simulink model "W06_city_highway_cs"  (R2019a)
settings: Solver=ode5  StartTime=0.0  StopTime=inf  FixedStep=1/60  RelTol=1e-3
PreLoadFcn:
  | mbxruntime.callbacks.PreLoadFcn(bdroot);
PostLoadFcn:
  | mbxruntime.callbacks.PostLoadFcn(bdroot);
InitFcn:
  | mbxruntime.callbacks.InitFcn(bdroot);
StartFcn:
  | mbxruntime.callbacks.StartFcn(bdroot);
StopFcn:
  | mbxruntime.callbacks.StopFcn(bdroot);
model workspace: external: MAT-File .\W06_city_highway_cs_hws.mat (data not in the file)
undefined symbols (not defined in the file or in its folder): DiscIntNeverNeededParam, FovAzimuth, FovAzimuthDefined, FovElevation, FovElevationDefined, Header, InitImageOutputDir, LocationX, LocationXDefined, LocationY, LocationYDefined, LocationZ, LocationZDefined, Orientation, OrientationPitch, OrientationPitchDefined, OrientationRoll, OrientationRollDefined, OrientationYaw, OrientationYawDefined, Poses, Poses_SL_Info, Position, W06_city_highway_cs_0270c22595f3b0e3, W06_city_highway_cs_086892688dd32ddc, W06_city_highway_cs_328c49ac39fca66b, W06_city_highway_cs_35ce05381b8ebe8c, W06_city_highway_cs_47b384f162638175, W06_city_highway_cs_766f76ce4de94dd5, W06_city_highway_cs_8c547f67cb81ffba, W06_city_highway_cs_aed52f2a7724a4f9, W06_city_highway_cs_Audi_A8_Sedan_1_Path_pathUniqueID, W06_city_highway_cs_b74cbb1f9f7331b5, W06_city_highway_cs_Citroen_C3_Hatchback_1_Path_pathUniqueID, W06_city_highway_cs_d395f8835e0c28b3, W06_city_highway_cs_e5f9d1759e19e2b4, W06_city_highway_cs_Toyota_Previa_MPV_1_Path_pathUniqueID
libraries: adeye_lib x26, simulink_extras x24, robotlib x7, sharedtransform x4, PreScanSimulinkLibrary x2, PreScanUsefulBlocks x1
(part 2 of 8)

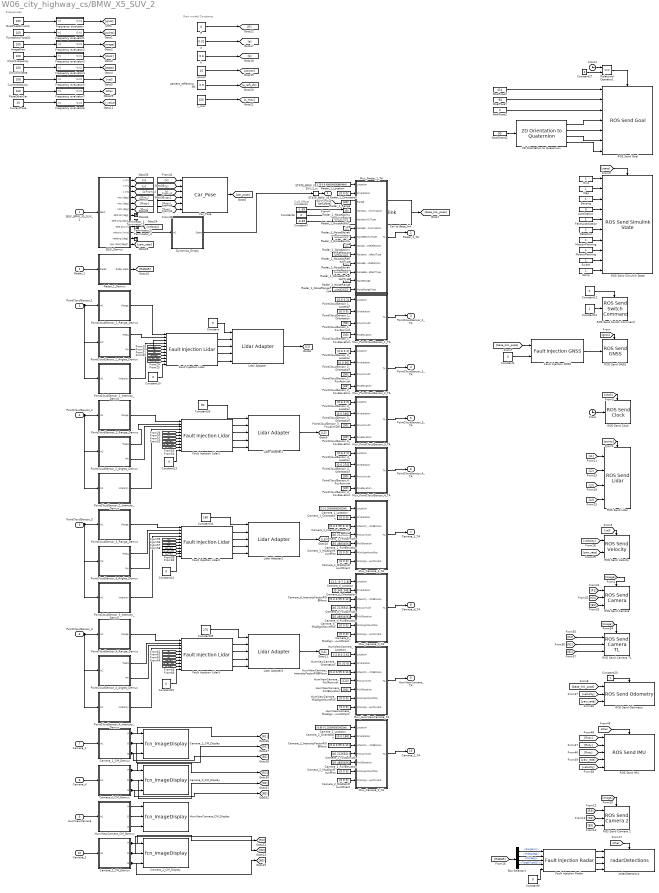
== system W06_city_highway_cs/BMW_X5_SUV_2 ==
  note: Frequencies
  note: CoG Offset
  note: Rain model Constants
  SELF_BMW_X5_SUV_2 : Inport  Tag=inport/SelfPort  OutDataTypeStr=Bus: PRESCAN_SELFSENSORDATA  PortDimensions=1  SampleTime=1/60  BusOutputAsStruct=on
  Radar_1 : Inport  Tag=inport/Radar  Port=2  OutDataTypeStr=Bus: PRESCAN_SCANNERSENSOR_MESSAGE  PortDimensions=7  SampleTime=1/20  BusOutputAsStruct=on
  PointCloudSensor_1 : Inport  Tag=inport/PointCloudInport  Port=3  OutDataTypeStr=single  SampleTime=1/20  BusOutputAsStruct=on
  PointCloudSensor_2 : Inport  Tag=inport/PointCloudInport  Port=4  OutDataTypeStr=single  SampleTime=1/20  BusOutputAsStruct=on
  PointCloudSensor_3 : Inport  Tag=inport/PointCloudInport  Port=5  OutDataTypeStr=single  SampleTime=1/20  BusOutputAsStruct=on
  PointCloudSensor_4 : Inport  Tag=inport/PointCloudInport  Port=6  OutDataTypeStr=single  SampleTime=1/20  BusOutputAsStruct=on
  Camera_1 : Inport  Tag=inport/Camera/CameraSensor  Port=7  OutDataTypeStr=uint8  SampleTime=1/20  BusOutputAsStruct=on
  Camera_tl : Inport  Tag=inport/Camera/CameraSensor  Port=8  OutDataTypeStr=uint8  SampleTime=1/20  BusOutputAsStruct=on
  HumViewCamera : Inport  Tag=inport/Camera/CameraSensor  Port=9  OutDataTypeStr=uint8  SampleTime=1/60  BusOutputAsStruct=on
  Camera_2 : Inport  Tag=inport/Camera/CameraSensor  Port=10  OutDataTypeStr=uint8  SampleTime=1/20  BusOutputAsStruct=on
  2D Orientation to Quaternion : adeye_lib/2D Orientation to Quaternion  SystemSampleTime=-1
  Bus Selector1 : BusSelector  OutputSignals=Range[m],Theta[deg],Phi[deg],TargetTypeID[-]
  Camera_1_CM_Demux : Subsystem  Tag=demux/Camera/Color  mask{SensorName=Camera_1, hres=960, vres=720}
      mask prompts: SensorName "Sensor Name"; hres "Horizontal Resolution"; vres "Vertical Resolution"
      mask Help: eval('openHelp(457)')
      mask Display:
      | fprintf('MONO CAMERA:\n Color\n %s \n %d x %d px',SensorName,hres,vres)
      | port_label('output',1,'R')
      | port_label('output',2,'G')
      | port_label('output',3,'B')
  Camera_1_CM_Display : M-S-Function  Tag=CameraSensor_Color_Display  InitFcn=InitImageOutputDir(gcb);  FunctionName=fcn_ImageDisplay  Parameters=SensorName EnableDisplay EnablePosition DisplayPosition FigureHandle SaveResults BitmapFormat TempOutputDir CameraType DataType  mask(PreScan Color Display Block){SensorName=Camera_1, EnableDisplay=on, EnablePosition=off, DisplayPosition=[10 10 960 720], FigureHandle=640605, SaveResults=off, Format=PNG, TempOutputDir=0, CameraType=Mono, DataType=uint8}
      mask prompts: SensorName "User Specified: Title of Display"; EnableDisplay "Active"; EnablePosition "Set Display window position"; DisplayPosition "Display window position [xpos ypos width height]"; FigureHandle "Unique Handle"; SaveResults "Save results"; TempOutputDir "OutputDir"; CameraType "Camera Type"; DataType "Image Data Type"
      mask help: This block displays the RGB output of a PreScan camera sensor.
      mask init:
      | if EnableDisplay
      |     EnableString='';
      |     EnableColor='gray';
      | else
      |     EnableString='INACTIVE';
      |     EnableColor='red';
      | end
      | switch Format
      |     case 1
      |         BitmapFormat = 'png';
      |     case 2
      |         BitmapFormat = 'bmp';
      |     case 3
      |         BitmapFormat = 'jpg';
      | end 
      | if CameraType==1
      |     CameraTypeName='MONO';
      |     PortNumber=0;
      | else
      |     CameraTypeName='STEREO';
      |     PortNumber=3;
      | end
      settings: CopyFcn=CopyFcnDisplay  DeleteFcn=PreScanBlockDeleteFcn;  ModelCloseFcn=fcn_ImageDisplay_ModelCloseFcn
      mask Help: eval('openHelp(457)')
      mask Callback EnablePosition:
      | MV=get_param(gcb,'MaskVisibilities');
      | if strcmp(get_param(gcb,'EnablePosition'),'on')
      |     MV{4}='on';
      | else
      |     MV{4}='off';
      | end
      | set_param(gcb,'MaskVisibilities',MV);
      | clear MV;
      mask TypeOptions Format: PNG | BMP | JPG
      mask TypeOptions CameraType: Mono | Stereo
      mask TypeOptions DataType: uint8 | single
      mask Display:
      | color(EnableColor);
      | fprintf('%s\n DISPLAY:\n Color \n %s',EnableString,SensorName)
      | port_label('input',1,'R')
      | port_label('input',2,'G')
      | port_label('input',3,'B')
      | port_label('input',PortNumber+1,'R')
      | port_label('input',PortNumber+2,'G')
      | port_label('input',PortNumber+3,'B')
  Camera_1_FoVAzimuth : Constant  Tag=Camera_1_FoVAzimuth  Value=[46.2126541]
  Camera_1_FoVElevation : Constant  Tag=Camera_1_FoVElevation  Value=[35.4893456]
  Camera_1_IntensityFactorRGBMono : Constant  Tag=Camera_1_IntensityFactorRGBMono  Value=[0.3 0.59 0.11]
  Camera_1_Location : Constant  Tag=Camera_1_Location  Value=[2 0 1.32000005245209]
  Camera_1_MisAlignMountOrient : Constant  Tag=Camera_1_MisAlignMountOrient  Value=[0 0 0]
  Camera_1_MisAlignMountPos : Constant  Tag=Camera_1_MisAlignMountPos  Value=[0 0 0]
  Camera_1_Orientation : Constant  Tag=Camera_1_Orientation  Value=[0 0 0]
  Camera_2_CM_Demux : Subsystem  Tag=demux/Camera/Color  mask{SensorName=Camera_2, hres=960, vres=720}
      mask prompts: SensorName "Sensor Name"; hres "Horizontal Resolution"; vres "Vertical Resolution"
      mask Help: eval('openHelp(457)')
      mask Display:
      | fprintf('MONO CAMERA:\n Color\n %s \n %d x %d px',SensorName,hres,vres)
      | port_label('output',1,'R')
      | port_label('output',2,'G')
      | port_label('output',3,'B')
  Camera_2_CM_Display : M-S-Function  Tag=CameraSensor_Color_Display  InitFcn=InitImageOutputDir(gcb);  FunctionName=fcn_ImageDisplay  Parameters=SensorName EnableDisplay EnablePosition DisplayPosition FigureHandle SaveResults BitmapFormat TempOutputDir CameraType DataType  mask(PreScan Color Display Block){SensorName=Camera_2, EnableDisplay=on, EnablePosition=off, DisplayPosition=[10 10 960 720], FigureHandle=640608, SaveResults=off, Format=PNG, TempOutputDir=0, CameraType=Mono, DataType=uint8}
      mask prompts: SensorName "User Specified: Title of Display"; EnableDisplay "Active"; EnablePosition "Set Display window position"; DisplayPosition "Display window position [xpos ypos width height]"; FigureHandle "Unique Handle"; SaveResults "Save results"; TempOutputDir "OutputDir"; CameraType "Camera Type"; DataType "Image Data Type"
      mask help: This block displays the RGB output of a PreScan camera sensor.
      mask init: same as W06_city_highway_cs/BMW_X5_SUV_2/Camera_1_CM_Display
      settings: CopyFcn=CopyFcnDisplay  DeleteFcn=PreScanBlockDeleteFcn;  ModelCloseFcn=fcn_ImageDisplay_ModelCloseFcn
      mask Help: eval('openHelp(457)')
      mask Callback EnablePosition:
      | MV=get_param(gcb,'MaskVisibilities');
      | if strcmp(get_param(gcb,'EnablePosition'),'on')
      |     MV{4}='on';
      | else
      |     MV{4}='off';
      | end
      | set_param(gcb,'MaskVisibilities',MV);
      | clear MV;
      mask TypeOptions Format: PNG | BMP | JPG
      mask TypeOptions CameraType: Mono | Stereo
      mask TypeOptions DataType: uint8 | single
      mask Display:
      | color(EnableColor);
      | fprintf('%s\n DISPLAY:\n Color \n %s',EnableString,SensorName)
      | port_label('input',1,'R')
      | port_label('input',2,'G')
      | port_label('input',3,'B')
      | port_label('input',PortNumber+1,'R')
      | port_label('input',PortNumber+2,'G')
      | port_label('input',PortNumber+3,'B')
  Camera_2_FoVAzimuth : Constant  Tag=Camera_2_FoVAzimuth  Value=[46.2126541]
  Camera_2_FoVElevation : Constant  Tag=Camera_2_FoVElevation  Value=[35.4893456]
  Camera_2_IntensityFactorRGBMono : Constant  Tag=Camera_2_IntensityFactorRGBMono  Value=[0.3 0.59 0.11]
  Camera_2_Location : Constant  Tag=Camera_2_Location  Value=[-0.95 0 1.32000005245209]
  Camera_2_MisAlignMountOrient : Constant  Tag=Camera_2_MisAlignMountOrient  Value=[0 0 0]
  Camera_2_MisAlignMountPos : Constant  Tag=Camera_2_MisAlignMountPos  Value=[0 0 0]
  Camera_2_Orientation : Constant  Tag=Camera_2_Orientation  Value=[0 0 180]
  Camera_tl_CM_Demux : Subsystem  Tag=demux/Camera/Color  mask{SensorName=Camera_tl, hres=960, vres=720}
      mask prompts: SensorName "Sensor Name"; hres "Horizontal Resolution"; vres "Vertical Resolution"
      mask Help: eval('openHelp(457)')
      mask Display:
      | fprintf('MONO CAMERA:\n Color\n %s \n %d x %d px',SensorName,hres,vres)
      | port_label('output',1,'R')
      | port_label('output',2,'G')
      | port_label('output',3,'B')
  Camera_tl_CM_Display : M-S-Function  Tag=CameraSensor_Color_Display  InitFcn=InitImageOutputDir(gcb);  FunctionName=fcn_ImageDisplay  Parameters=SensorName EnableDisplay EnablePosition DisplayPosition FigureHandle SaveResults BitmapFormat TempOutputDir CameraType DataType  mask(PreScan Color Display Block){SensorName=Camera_tl, EnableDisplay=on, EnablePosition=off, DisplayPosition=[10 10 960 720], FigureHandle=640606, SaveResults=off, Format=PNG, TempOutputDir=0, CameraType=Mono, DataType=uint8}
      mask prompts: SensorName "User Specified: Title of Display"; EnableDisplay "Active"; EnablePosition "Set Display window position"; DisplayPosition "Display window position [xpos ypos width height]"; FigureHandle "Unique Handle"; SaveResults "Save results"; TempOutputDir "OutputDir"; CameraType "Camera Type"; DataType "Image Data Type"
      mask help: This block displays the RGB output of a PreScan camera sensor.
      mask init: same as W06_city_highway_cs/BMW_X5_SUV_2/Camera_1_CM_Display
      settings: CopyFcn=CopyFcnDisplay  DeleteFcn=PreScanBlockDeleteFcn;  ModelCloseFcn=fcn_ImageDisplay_ModelCloseFcn
      mask Help: eval('openHelp(457)')
      mask Callback EnablePosition:
      | MV=get_param(gcb,'MaskVisibilities');
      | if strcmp(get_param(gcb,'EnablePosition'),'on')
      |     MV{4}='on';
      | else
      |     MV{4}='off';
      | end
      | set_param(gcb,'MaskVisibilities',MV);
      | clear MV;
      mask TypeOptions Format: PNG | BMP | JPG
      mask TypeOptions CameraType: Mono | Stereo
      mask TypeOptions DataType: uint8 | single
      mask Display:
      | color(EnableColor);
      | fprintf('%s\n DISPLAY:\n Color \n %s',EnableString,SensorName)
      | port_label('input',1,'R')
      | port_label('input',2,'G')
      | port_label('input',3,'B')
      | port_label('input',PortNumber+1,'R')
      | port_label('input',PortNumber+2,'G')
      | port_label('input',PortNumber+3,'B')
  Camera_tl_FoVAzimuth : Constant  Tag=Camera_tl_FoVAzimuth  Value=[46.2126541]
  Camera_tl_FoVElevation : Constant  Tag=Camera_tl_FoVElevation  Value=[35.4893456]
  Camera_tl_IntensityFactorRGBMono : Constant  Tag=Camera_tl_IntensityFactorRGBMono  Value=[0.3 0.59 0.11]
  Camera_tl_Location : Constant  Tag=Camera_tl_Location  Value=[1.1 -0.7 1.8]
  Camera_tl_MisAlignMountOrient : Constant  Tag=Camera_tl_MisAlignMountOrient  Value=[0 0 0]
  Camera_tl_MisAlignMountPos : Constant  Tag=Camera_tl_MisAlignMountPos  Value=[0 0 0]
  Camera_tl_Orientation : Constant  Tag=Camera_tl_Orientation  Value=[0 345 345]
  Car to Base_link : adeye_lib/Car to Base_link  SystemSampleTime=-1
  Car_Pose : adeye_lib/Car_Pose  SystemSampleTime=-1
  Clock : Clock
  Clock2 : Clock
  ClockFrequency : Constant  Value=100
  Constant{,10,13..15} (5 alike) : Constant  Value=0  OutDataTypeStr=Inherit: Inherit via back propagation
  Constant1 : Constant  Value=0  OutDataTypeStr=Inherit: Inherit via back propagation  SampleTime=0.05
  Constant11 : Constant  OutDataTypeStr=Inherit: Inherit via back propagation  SampleTime=0.05
  Constant12 : Constant  Value=0  OutDataTypeStr=Inherit: Inherit via back propagation  SampleTime=0.05
  Constant2 : Constant  Value=-1.69
  Constant20 : Constant
  Constant27 : Constant  Value=0
  Constant33 : Constant  Value=90  OutDataTypeStr=Inherit: Inherit via back propagation
  Constant34 : Constant  Value=180  OutDataTypeStr=Inherit: Inherit via back propagation
  Constant35 : Constant  Value=270  OutDataTypeStr=Inherit: Inherit via back propagation
  Constant6 : Constant  Value=0
  Constant7 : Constant  Value=-0.69
  Constant9 : Constant  Value=0
  CurrentPose : Constant  Value=10
  CurrentVelocity : Constant  Value=100
  Detection : Constant
  Dynamics_Empty : Subsystem  Tag=Dynamics_Empty
      mask Help: eval('openHelp(202)')
      mask Display: port_label('output', 1, 'State');text(0,0,' Empty\n')
  FakeLocalization : Constant
  Fault Injection GNSS : adeye_lib/Fault Injection GNSS  v=0.0001  f=20
  Fault Injection Lidar{,1..3} (4 alike) : adeye_lib/Fault Injection Lidar  vr=0.0001  vi=0.0001  f=20  p=225*16
  Fault Injection Radar : adeye_lib/Fault Injection Radar  n=7  vr=1  vt=1  vp=1
  Frequency evaluator : Subsystem
  Frequency evaluator1 : Subsystem
  Frequency evaluator2 : Subsystem
  Frequency evaluator3 : Subsystem
  Frequency evaluator4 : Subsystem
  Frequency evaluator5 : Subsystem
  Frequency evaluator6 : Subsystem
  Frequency evaluator7 : Subsystem
  GnssPoseSimulink : Constant  Value=100
  GoalOrientZ : Constant  Value=90
  GoalPoseX : Constant  Value=414
  GoalPoseY : Constant  Value=-83
  GoalPoseZ : Constant  Value=0
  HumViewCamera_CM_Demux : Subsystem  Tag=demux/Camera/Color  mask{SensorName=HumViewCamera, hres=1871, vres=1080}
      mask prompts: SensorName "Sensor Name"; hres "Horizontal Resolution"; vres "Vertical Resolution"
      mask Help: eval('openHelp(457)')
      mask Display:
      | fprintf('MONO CAMERA:\n Color\n %s \n %d x %d px',SensorName,hres,vres)
      | port_label('output',1,'R')
      | port_label('output',2,'G')
      | port_label('output',3,'B')
  HumViewCamera_CM_Display : M-S-Function  Tag=CameraSensor_Color_Display  InitFcn=InitImageOutputDir(gcb);  FunctionName=fcn_ImageDisplay  Parameters=SensorName EnableDisplay EnablePosition DisplayPosition FigureHandle SaveResults BitmapFormat TempOutputDir CameraType DataType  mask(PreScan Color Display Block){SensorName=HumViewCamera, EnableDisplay=on, EnablePosition=off, DisplayPosition=[10 10 1871 1080], FigureHandle=640607, SaveResults=off, Format=PNG, TempOutputDir=0, CameraType=Mono, DataType=uint8}
      mask prompts: SensorName "User Specified: Title of Display"; EnableDisplay "Active"; EnablePosition "Set Display window position"; DisplayPosition "Display window position [xpos ypos width height]"; FigureHandle "Unique Handle"; SaveResults "Save results"; TempOutputDir "OutputDir"; CameraType "Camera Type"; DataType "Image Data Type"
      mask help: This block displays the RGB output of a PreScan camera sensor.
      mask init: same as W06_city_highway_cs/BMW_X5_SUV_2/Camera_1_CM_Display
      settings: CopyFcn=CopyFcnDisplay  DeleteFcn=PreScanBlockDeleteFcn;  ModelCloseFcn=fcn_ImageDisplay_ModelCloseFcn
      mask Help: eval('openHelp(457)')
      mask Callback EnablePosition:
      | MV=get_param(gcb,'MaskVisibilities');
      | if strcmp(get_param(gcb,'EnablePosition'),'on')
      |     MV{4}='on';
      | else
      |     MV{4}='off';
      | end
      | set_param(gcb,'MaskVisibilities',MV);
      | clear MV;
      mask TypeOptions Format: PNG | BMP | JPG
      mask TypeOptions CameraType: Mono | Stereo
      mask TypeOptions DataType: uint8 | single
      mask Display:
      | color(EnableColor);
      | fprintf('%s\n DISPLAY:\n Color \n %s',EnableString,SensorName)
      | port_label('input',1,'R')
      | port_label('input',2,'G')
      | port_label('input',3,'B')
      | port_label('input',PortNumber+1,'R')
      | port_label('input',PortNumber+2,'G')
      | port_label('input',PortNumber+3,'B')
  HumViewCamera_FoVAzimuth : Constant  Tag=HumViewCamera_FoVAzimuth  Value=[120]
  HumViewCamera_FoVElevation : Constant  Tag=HumViewCamera_FoVElevation  Value=[90]
  HumViewCamera_IntensityFactorRGBMono : Constant  Tag=HumViewCamera_IntensityFactorRGBMono  Value=[0.3 0.59 0.11]
  HumViewCamera_Location : Constant  Tag=HumViewCamera_Location  Value=[-2.8 0 2.6]
  HumViewCamera_MisAlignMountOrient : Constant  Tag=HumViewCamera_MisAlignMountOrient  Value=[0 0 0]
  HumViewCamera_MisAlignMountPos : Constant  Tag=HumViewCamera_MisAlignMountPos  Value=[0 0 0]
  HumViewCamera_Orientation : Constant  Tag=HumViewCamera_Orientation  Value=[0 31 0]
  ImageRaw : Constant  Value=100
  Lidar Adapter{,1..3} (4 alike) : adeye_lib/Lidar Adapter  SystemSampleTime=-1
  Localization : Constant  Value=0
  Map : Constant
  MissionPlanning : Constant
  MotionPlanning : Constant
  Mux_Camera_1_TA : Subsystem  Tag=mux/Camera_TA/CameraSensor
  Mux_Camera_2_TA : Subsystem  Tag=mux/Camera_TA/CameraSensor
  Mux_Camera_tl_TA : Subsystem  Tag=mux/Camera_TA/CameraSensor
  Mux_HumViewCamera_TA : Subsystem  Tag=mux/Camera_TA/CameraSensor
  Mux_PointCloudSensor_1_TA : Subsystem  Tag=mux/SensorTA
  Mux_PointCloudSensor_2_TA : Subsystem  Tag=mux/SensorTA
  Mux_PointCloudSensor_3_TA : Subsystem  Tag=mux/SensorTA
  Mux_PointCloudSensor_4_TA : Subsystem  Tag=mux/SensorTA
  Mux_Radar_1_TA : Subsystem  Tag=mux/Radar_TA
  PointCloudSensor_1_Angles_Demux : Subsystem  Tag=demux/PCS/Angles  mask{SensorName=PointCloudSensor_1, offset=225, hres=225, vres=16}
      mask prompts: SensorName "Sensor Name"; offset "Data Start"; hres "Horizontal Resolution"; vres "Vertical Resolution"
      mask Help: eval('openHelp(6400)')
      mask Display:
      | fprintf('Point Cloud:\n Data\n %s \n %d x %d px',SensorName,hres,vres)
      | port_label('output',1,'Theta')
      | port_label('output',2,'Phi')
  PointCloudSensor_1_FovAzimuth : Constant  Tag=PointCloudSensor_1_FovAzimuth  Value=[90]
  PointCloudSensor_1_FovElevation : Constant  Tag=PointCloudSensor_1_FovElevation  Value=[30]
  PointCloudSensor_1_Intensity_Demux : Subsystem  Tag=demux/PCS/Intensity  mask{SensorName=PointCloudSensor_1, offset=675, hres=225, vres=16}
      mask prompts: SensorName "Sensor Name"; offset "Data Start"; hres "Horizontal Resolution"; vres "Vertical Resolution"
      mask Help: eval('openHelp(6400)')
      mask Display:
      | fprintf('Point Cloud:\n Data\n %s \n %d x %d px',SensorName,hres,vres)
      | port_label('output',1,'Intensity')
  PointCloudSensor_1_Location : Constant  Tag=PointCloudSensor_1_Location  Value=[0.6 0 2]
  PointCloudSensor_1_Orientation : Constant  Tag=PointCloudSensor_1_Orientation  Value=[0 0 0]
  PointCloudSensor_1_Range_Demux : Subsystem  Tag=demux/PCS/Range  mask{SensorName=PointCloudSensor_1, offset=0, hres=225, vres=16}
      mask prompts: SensorName "Sensor Name"; offset "Data Start"; hres "Horizontal Resolution"; vres "Vertical Resolution"
      mask Help: eval('openHelp(6400)')
      mask Display:
      | fprintf('Point Cloud:\n Data\n %s \n %d x %d px',SensorName,hres,vres)
      | port_label('output',1,'Range')
  PointCloudSensor_2_Angles_Demux : Subsystem  Tag=demux/PCS/Angles  mask{SensorName=PointCloudSensor_2, offset=225, hres=225, vres=16}
      mask prompts: SensorName "Sensor Name"; offset "Data Start"; hres "Horizontal Resolution"; vres "Vertical Resolution"
      mask Help: eval('openHelp(6400)')
      mask Display:
      | fprintf('Point Cloud:\n Data\n %s \n %d x %d px',SensorName,hres,vres)
      | port_label('output',1,'Theta')
      | port_label('output',2,'Phi')
  PointCloudSensor_2_FovAzimuth : Constant  Tag=PointCloudSensor_2_FovAzimuth  Value=[90]
  PointCloudSensor_2_FovElevation : Constant  Tag=PointCloudSensor_2_FovElevation  Value=[30]
  PointCloudSensor_2_Intensity_Demux : Subsystem  Tag=demux/PCS/Intensity  mask{SensorName=PointCloudSensor_2, offset=675, hres=225, vres=16}
      mask prompts: SensorName "Sensor Name"; offset "Data Start"; hres "Horizontal Resolution"; vres "Vertical Resolution"
      mask Help: eval('openHelp(6400)')
      mask Display:
      | fprintf('Point Cloud:\n Data\n %s \n %d x %d px',SensorName,hres,vres)
      | port_label('output',1,'Intensity')
  PointCloudSensor_2_Location : Constant  Tag=PointCloudSensor_2_Location  Value=[0.6 0 2]
  PointCloudSensor_2_Orientation : Constant  Tag=PointCloudSensor_2_Orientation  Value=[0 0 90]
  PointCloudSensor_2_Range_Demux : Subsystem  Tag=demux/PCS/Range  mask{SensorName=PointCloudSensor_2, offset=0, hres=225, vres=16}
      mask prompts: SensorName "Sensor Name"; offset "Data Start"; hres "Horizontal Resolution"; vres "Vertical Resolution"
      mask Help: eval('openHelp(6400)')
      mask Display:
      | fprintf('Point Cloud:\n Data\n %s \n %d x %d px',SensorName,hres,vres)
      | port_label('output',1,'Range')
  PointCloudSensor_3_Angles_Demux : Subsystem  Tag=demux/PCS/Angles  mask{SensorName=PointCloudSensor_3, offset=225, hres=225, vres=16}
      mask prompts: SensorName "Sensor Name"; offset "Data Start"; hres "Horizontal Resolution"; vres "Vertical Resolution"
      mask Help: eval('openHelp(6400)')
      mask Display:
      | fprintf('Point Cloud:\n Data\n %s \n %d x %d px',SensorName,hres,vres)
      | port_label('output',1,'Theta')
      | port_label('output',2,'Phi')
  PointCloudSensor_3_FovAzimuth : Constant  Tag=PointCloudSensor_3_FovAzimuth  Value=[90]
  PointCloudSensor_3_FovElevation : Constant  Tag=PointCloudSensor_3_FovElevation  Value=[30]
  PointCloudSensor_3_Intensity_Demux : Subsystem  Tag=demux/PCS/Intensity  mask{SensorName=PointCloudSensor_3, offset=675, hres=225, vres=16}
      mask prompts: SensorName "Sensor Name"; offset "Data Start"; hres "Horizontal Resolution"; vres "Vertical Resolution"
      mask Help: eval('openHelp(6400)')
      mask Display:
      | fprintf('Point Cloud:\n Data\n %s \n %d x %d px',SensorName,hres,vres)
      | port_label('output',1,'Intensity')
  PointCloudSensor_3_Location : Constant  Tag=PointCloudSensor_3_Location  Value=[0.6 0 2]
  PointCloudSensor_3_Orientation : Constant  Tag=PointCloudSensor_3_Orientation  Value=[0 0 180]
  PointCloudSensor_3_Range_Demux : Subsystem  Tag=demux/PCS/Range  mask{SensorName=PointCloudSensor_3, offset=0, hres=225, vres=16}
      mask prompts: SensorName "Sensor Name"; offset "Data Start"; hres "Horizontal Resolution"; vres "Vertical Resolution"
      mask Help: eval('openHelp(6400)')
      mask Display:
      | fprintf('Point Cloud:\n Data\n %s \n %d x %d px',SensorName,hres,vres)
      | port_label('output',1,'Range')
  PointCloudSensor_4_Angles_Demux : Subsystem  Tag=demux/PCS/Angles  mask{SensorName=PointCloudSensor_4, offset=225, hres=225, vres=16}
      mask prompts: SensorName "Sensor Name"; offset "Data Start"; hres "Horizontal Resolution"; vres "Vertical Resolution"
      mask Help: eval('openHelp(6400)')
      mask Display:
      | fprintf('Point Cloud:\n Data\n %s \n %d x %d px',SensorName,hres,vres)
      | port_label('output',1,'Theta')
      | port_label('output',2,'Phi')
  PointCloudSensor_4_FovAzimuth : Constant  Tag=PointCloudSensor_4_FovAzimuth  Value=[90]
  PointCloudSensor_4_FovElevation : Constant  Tag=PointCloudSensor_4_FovElevation  Value=[30]
  PointCloudSensor_4_Intensity_Demux : Subsystem  Tag=demux/PCS/Intensity  mask{SensorName=PointCloudSensor_4, offset=675, hres=225, vres=16}
      mask prompts: SensorName "Sensor Name"; offset "Data Start"; hres "Horizontal Resolution"; vres "Vertical Resolution"
      mask Help: eval('openHelp(6400)')
      mask Display:
      | fprintf('Point Cloud:\n Data\n %s \n %d x %d px',SensorName,hres,vres)
      | port_label('output',1,'Intensity')
  PointCloudSensor_4_Location : Constant  Tag=PointCloudSensor_4_Location  Value=[0.6 0 2]
  PointCloudSensor_4_Orientation : Constant  Tag=PointCloudSensor_4_Orientation  Value=[0 0 270]
  PointCloudSensor_4_Range_Demux : Subsystem  Tag=demux/PCS/Range  mask{SensorName=PointCloudSensor_4, offset=0, hres=225, vres=16}
      mask prompts: SensorName "Sensor Name"; offset "Data Start"; hres "Horizontal Resolution"; vres "Vertical Resolution"
      mask Help: eval('openHelp(6400)')
      mask Display:
      | fprintf('Point Cloud:\n Data\n %s \n %d x %d px',SensorName,hres,vres)
      | port_label('output',1,'Range')
  PointsRawFloat32 : Constant  Value=100
  PoseOtherCar : Constant  Value=100
  R : Constant  Value=0
  ROS Send Camera : adeye_lib/ROS Send Camera  SystemSampleTime=-1
  ROS Send Camera 2 : adeye_lib/ROS Send Camera 2  SystemSampleTime=-1
  ROS Send Camera TL : adeye_lib/ROS Send Camera TL  SystemSampleTime=-1
  ROS Send Clock : adeye_lib/ROS Send Clock  SystemSampleTime=-1
  ROS Send GNSS : adeye_lib/ROS Send GNSS  SystemSampleTime=-1
  ROS Send Goal : adeye_lib/ROS Send Goal  SystemSampleTime=-1
  ROS Send IMU : adeye_lib/ROS Send IMU  SystemSampleTime=-1
  ROS Send Lidar : adeye_lib/ROS Send Lidar  SystemSampleTime=-1
  ROS Send Odometry : adeye_lib/ROS Send Odometry  SystemSampleTime=-1
  ROS Send Simulink State : adeye_lib/ROS Send Simulink State  SystemSampleTime=-1
  ROS Send Switch Command : adeye_lib/ROS Send Switch Command  SystemSampleTime=-1
  ROS Send Velocity : adeye_lib/ROS Send Velocity  SystemSampleTime=-1
  Radar_1_Demux : Subsystem  Tag=demux/Radar  TreatAsAtomicUnit=on  mask(PreScan Demux Block: Radar){MAXMESSAGES=7}
      mask prompts: MAXMESSAGES "Number of Objects"
      mask help:
      | The Radar Sensor is a detailed sensor based on a physical radar
      | model that includes Antenna GAIN Maps (AGM) and atmospheric
      | attenuation.
      |
      | For more information, please click Help.
      mask Help: eval('openHelp(1464)')
      mask Display:
      | port_label('input',1,'Radar')
      | port_label('output',1,'Radar Data')
  Radar_1_Location : Constant  Tag=Radar_1_Location  Value=[3.75 0 0.400000005960464]
  Radar_1_NoiseAziIlluType : Constant  Tag=Radar_1_NoiseAziIlluType  Value=uint32([0])
  Radar_1_NoiseAziReflectType : Constant  Tag=Radar_1_NoiseAziReflectType  Value=uint32([0])
  Radar_1_NoiseAzimuthIllumination : Constant  Tag=Radar_1_NoiseAzimuthIllumination  Value=[0]
  Radar_1_NoiseAzimuthReflection : Constant  Tag=Radar_1_NoiseAzimuthReflection  Value=[0]
  Radar_1_NoiseElevIlluType : Constant  Tag=Radar_1_NoiseElevIlluType  Value=uint32([0])
  Radar_1_NoiseElevReflectType : Constant  Tag=Radar_1_NoiseElevReflectType  Value=uint32([0])
  Radar_1_NoiseElevationIllumination : Constant  Tag=Radar_1_NoiseElevationIllumination  Value=[0]
  Radar_1_NoiseElevationReflection : Constant  Tag=Radar_1_NoiseElevationReflection  Value=[0]
  Radar_1_NoiseRange : Constant  Tag=Radar_1_NoiseRange  Value=[0]
  Radar_1_NoiseRangeType : Constant  Tag=Radar_1_NoiseRangeType  Value=uint32([1])
  Radar_1_Orientation : Constant  Tag=Radar_1_Orientation  Value=[0 0 0]
  Radar_1_Range : Constant  Tag=Radar_1_Range  Value=[30]
  Relational Operator1 : RelationalOperator  Operator===  OutDataTypeStr=boolean  RndMeth=Simplest
  Rviz : Constant
  SELF_Demux : Subsystem  Tag=demux/SelfPort  mask(PreScan Demux Block:){}
      mask help:
      | The SELF port shows (state) information of the actor itself. The outputs are position in the experiment's axis system and the GPS coordinates, and the object's absolute velocity and compass heading.
      |
      | For more information, please click Help.
      settings: DeleteFcn=PreScanBlockDeleteFcn;
      mask Help: eval('openHelp(462)')
      mask Display:
      | port_label('output',1,'x [m]')
      | port_label('output',2,'y [m]')
      | port_label('output',3,'z [m]','texmode','on')
      | port_label('output',4,'Rotx [deg]','texmode','on')
      | port_label('output',5,'Roty [deg]','texmode','on')
      | port_label('output',6,'Rotz [deg]','texmode','on')
      | port_label('output',7,'GPS lat [deg]','texmode','on')
      | port_label('output',8,'GPS long [deg]','texmode','on')
      | port_label('output',9,'GPS alt [m]','texmode','on')
      | port_label('output',10,'Velocity [m/s]')
      | port_label('output',11,'Heading [deg]')
      | port_label('output',12,'Yaw rate [deg/s]')
  STATE_BMW_X5_SUV_2_rc : RateTransition  Tag=mux_rc/StatePort  OutPortSampleTimeOpt=Inherit
  Sensing : Constant
  SimulinkState : Constant  Value=100
  Ssmp : Constant
  Switch : Constant
  Terminator_{1..4} (4 alike) : Terminator
  a : Constant  Value=0.01
  b : Constant  Value=0.6
  percent_reflecting_sfc : Constant  Value=0.9
  power : Constant  Value=15
  radarDetections : adeye_lib/radarDetections  SystemSampleTime=-1
  z_max : Constant  Value=150
  STATE_BMW_X5_SUV_2_bus : Outport  Tag=outport/StatePort  OutDataTypeStr=Bus: PRESCAN_STATEACTUATORDATA  PortDimensions=1  SampleTime=1/60
  Radar_1_TA : Outport  Tag=outport/Radar_TA  Port=2  OutDataTypeStr=Bus: PRESCAN_SCANNERSENSOR_TA  PortDimensions=1  SampleTime=1/60
  PointCloudSensor_1_TA : Outport  Tag=outport/SensorTA  Port=3  OutDataTypeStr=Bus: PRESCAN_PCS_TA_DATA  PortDimensions=1  SampleTime=1/60
  PointCloudSensor_2_TA : Outport  Tag=outport/SensorTA  Port=4  OutDataTypeStr=Bus: PRESCAN_PCS_TA_DATA  PortDimensions=1  SampleTime=1/60
  PointCloudSensor_3_TA : Outport  Tag=outport/SensorTA  Port=5  OutDataTypeStr=Bus: PRESCAN_PCS_TA_DATA  PortDimensions=1  SampleTime=1/60
  PointCloudSensor_4_TA : Outport  Tag=outport/SensorTA  Port=6  OutDataTypeStr=Bus: PRESCAN_PCS_TA_DATA  PortDimensions=1  SampleTime=1/60
  Camera_1_TA : Outport  Tag=outport/Camera_TA/CameraSensor  Port=7  OutDataTypeStr=Bus: PRESCAN_CAMERASENSOR_TA  PortDimensions=1  SampleTime=1/60
  Camera_tl_TA : Outport  Tag=outport/Camera_TA/CameraSensor  Port=8  OutDataTypeStr=Bus: PRESCAN_CAMERASENSOR_TA  PortDimensions=1  SampleTime=1/60
  HumViewCamera_TA : Outport  Tag=outport/Camera_TA/CameraSensor  Port=9  OutDataTypeStr=Bus: PRESCAN_CAMERASENSOR_TA  PortDimensions=1  SampleTime=1/60
  Camera_2_TA : Outport  Tag=outport/Camera_TA/CameraSensor  Port=10  OutDataTypeStr=Bus: PRESCAN_CAMERASENSOR_TA  PortDimensions=1  SampleTime=1/60
  tag scope: other=global, x_value=global
  wires:
  Camera_1_CM_Demux/1(R) -> [R1], Camera_1_CM_Display/1
  Camera_1_CM_Demux/2(G) -> [G1], Camera_1_CM_Display/2
  Camera_1_CM_Demux/3(B) -> [B1], Camera_1_CM_Display/3
  Camera_tl_CM_Demux/1(R) -> [R2], Camera_tl_CM_Display/1
  Camera_tl_CM_Demux/2(G) -> [G2], Camera_tl_CM_Display/2
  Camera_tl_CM_Demux/3(B) -> [B2], Camera_tl_CM_Display/3
  Camera_2_CM_Demux/1(R) -> [R3], Camera_2_CM_Display/1
  Camera_2_CM_Demux/2(G) -> [G3], Camera_2_CM_Display/2
  Camera_2_CM_Demux/3(B) -> [B3], Camera_2_CM_Display/3
  Radar_1_Demux/1(Radar Data) -> [RADAR]
  SELF_Demux/1(x [m]) -> [x]
  SELF_Demux/2(y [m]) -> [y]
  SELF_Demux/3(z [m]) -> [z]
  SELF_Demux/4(rotx [deg]) -> [Rotx]
  SELF_Demux/5(roty [deg]) -> [Roty]
  SELF_Demux/6(rotz [deg]) -> [Rotz]
  SELF_Demux/12(yaw rate [deg/s]) -> [yaw_rate]
  ClockFrequency/1 -> Frequency evaluator3/1(In1)
  Frequency evaluator5/1(Out1) -> [vel]
  CurrentPose/1 -> Frequency evaluator6/1(In1)
  PoseOtherCar/1 -> Frequency evaluator7/1(In1)
  PointsRawFloat32/1 -> Frequency evaluator1/1(In1)
  Frequency evaluator3/1(Out1) -> [clock]
  Frequency evaluator6/1(Out1) -> [x_value]
  SimulinkState/1 -> Frequency evaluator4/1(In1)
  Frequency evaluator1/1(Out1) -> [points]
  ImageRaw/1 -> Frequency evaluator2/1(In1)
  GnssPoseSimulink/1 -> Frequency evaluator/1(In1)
  Frequency evaluator2/1(Out1) -> [image]
  Frequency evaluator4/1(Out1) -> [state]
  CurrentVelocity/1 -> Frequency evaluator5/1(In1)
  Frequency evaluator7/1(Out1) -> [other]
  Frequency evaluator/1(Out1) -> [gnss]
  [z] -> Car_Pose/3
  [Roty] -> Car_Pose/5
  [Rotx] -> Car_Pose/4
  [y] -> Car_Pose/2
  [Rotz] -> Car_Pose/6
  [x] -> Car_Pose/1
  Car_Pose/1 -> [car_pose]
  SELF_Demux/10(velocity [m/s]) -> [velocity], Dynamics_Empty/1(In1)
  PointCloudSensor_1_Range_Demux/1(Range) -> Fault Injection Lidar/1
  PointCloudSensor_1_Angles_Demux/1(Theta) -> Fault Injection Lidar/2
  PointCloudSensor_1_Angles_Demux/2(Phi) -> Fault Injection Lidar/3
  PointCloudSensor_1_Intensity_Demux/1(Intensity) -> Fault Injection Lidar/4
  [b] -> Fault Injection Lidar/7
  [p_refl_sfc] -> Fault Injection Lidar/9
  [power] -> Fault Injection Lidar/8
  [a] -> Fault Injection Lidar/6
  Constant10/1 -> Fault Injection Lidar/11
  [z_max] -> Fault Injection Lidar/10
  [R] -> Fault Injection Lidar/5
  Fault Injection Lidar/2 -> Lidar Adapter/3
  Fault Injection Lidar/3 -> Lidar Adapter/4
  Fault Injection Lidar/1 -> Lidar Adapter/2
  Lidar Adapter/1 -> [L1]
  Fault Injection Lidar/4 -> Lidar Adapter/5
  Constant/1 -> Lidar Adapter/1
  Fault Injection Lidar1/3 -> Lidar Adapter1/4
  [z_max] -> Fault Injection Lidar1/10
  [power] -> Fault Injection Lidar1/8
  Constant33/1 -> Lidar Adapter1/1
  Fault Injection Lidar1/1 -> Lidar Adapter1/2
  [R] -> Fault Injection Lidar1/5
  [a] -> Fault Injection Lidar1/6
  Constant13/1 -> Fault Injection Lidar1/11
  [p_refl_sfc] -> Fault Injection Lidar1/9
  [b] -> Fault Injection Lidar1/7
  PointCloudSensor_2_Angles_Demux/1(Theta) -> Fault Injection Lidar1/2
  PointCloudSensor_2_Angles_Demux/2(Phi) -> Fault Injection Lidar1/3
  Fault Injection Lidar1/4 -> Lidar Adapter1/5
  Lidar Adapter1/1 -> [L2]
  PointCloudSensor_2_Intensity_Demux/1(Intensity) -> Fault Injection Lidar1/4
  PointCloudSensor_2_Range_Demux/1(Range) -> Fault Injection Lidar1/1
  Fault Injection Lidar1/2 -> Lidar Adapter1/3
  Fault Injection Lidar2/3 -> Lidar Adapter2/4
  Fault Injection Lidar2/1 -> Lidar Adapter2/2
  [b] -> Fault Injection Lidar2/7
  Constant14/1 -> Fault Injection Lidar2/11
  [z_max] -> Fault Injection Lidar2/10
  [R] -> Fault Injection Lidar2/5
  PointCloudSensor_3_Angles_Demux/1(Theta) -> Fault Injection Lidar2/2
  [p_refl_sfc] -> Fault Injection Lidar2/9
  PointCloudSensor_3_Intensity_Demux/1(Intensity) -> Fault Injection Lidar2/4
  Constant34/1 -> Lidar Adapter2/1
  [a] -> Fault Injection Lidar2/6
  [power] -> Fault Injection Lidar2/8
  PointCloudSensor_3_Range_Demux/1(Range) -> Fault Injection Lidar2/1
  Lidar Adapter2/1 -> [L3]
  Fault Injection Lidar2/4 -> Lidar Adapter2/5
  Fault Injection Lidar2/2 -> Lidar Adapter2/3
  PointCloudSensor_3_Angles_Demux/2(Phi) -> Fault Injection Lidar2/3
  Lidar Adapter3/1 -> [L4]
  Fault Injection Lidar3/1 -> Lidar Adapter3/2
  [z_max] -> Fault Injection Lidar3/10
  [power] -> Fault Injection Lidar3/8
  [b] -> Fault Injection Lidar3/7
  Fault Injection Lidar3/2 -> Lidar Adapter3/3
  Fault Injection Lidar3/3 -> Lidar Adapter3/4
  Fault Injection Lidar3/4 -> Lidar Adapter3/5
  Constant15/1 -> Fault Injection Lidar3/11
  PointCloudSensor_4_Angles_Demux/1(Theta) -> Fault Injection Lidar3/2
  Constant35/1 -> Lidar Adapter3/1
  [R] -> Fault Injection Lidar3/5
  PointCloudSensor_4_Angles_Demux/2(Phi) -> Fault Injection Lidar3/3
  [p_refl_sfc] -> Fault Injection Lidar3/9
  PointCloudSensor_4_Intensity_Demux/1(Intensity) -> Fault Injection Lidar3/4
  [a] -> Fault Injection Lidar3/6
  PointCloudSensor_4_Range_Demux/1(Range) -> Fault Injection Lidar3/1
  Constant6/1 -> Car to Base_link/3
  [car_pose] -> Car to Base_link/1
  Constant7/1 -> Car to Base_link/4
  Car to Base_link/1 -> [base_link_pose]
  Constant2/1 -> Car to Base_link/2
  z_max/1 -> [z_max]
  power/1 -> [power]
  percent_reflecting_sfc/1 -> [p_refl_sfc]
  a/1 -> [a]
  b/1 -> [b]
  R/1 -> [R]
  [state] -> ROS Send Simulink State/Enable
  GoalPoseY/1 -> ROS Send Goal/2
  [base_link_pose] -> Fault Injection GNSS/1
  MissionPlanning/1 -> ROS Send Simulink State/7
  Constant12/1 -> ROS Send Switch Command/Enable
  Rviz/1 -> ROS Send Simulink State/1
  Constant11/1 -> ROS Send Switch Command/1
  Clock2/1 -> Relational Operator1/1
  Ssmp/1 -> ROS Send Simulink State/10
  Constant1/1 -> Fault Injection GNSS/2
  GoalPoseZ/1 -> ROS Send Goal/3
  Fault Injection GNSS/1 -> ROS Send GNSS/1
  FakeLocalization/1 -> ROS Send Simulink State/5
  [gnss] -> ROS Send GNSS/Enable
  Map/1 -> ROS Send Simulink State/2
  Localization/1 -> ROS Send Simulink State/4
  Relational Operator1/1 -> ROS Send Goal/Enable
  Constant27/1 -> Relational Operator1/2
  GoalPoseX/1 -> ROS Send Goal/1
  Detection/1 -> ROS Send Simulink State/6
  Switch/1 -> ROS Send Simulink State/9
  MotionPlanning/1 -> ROS Send Simulink State/8
  Sensing/1 -> ROS Send Simulink State/3
  [G3] -> ROS Send Camera 2/2
  [Roty] -> ROS Send IMU/2
  Bus Selector1/4 -> Fault Injection Radar/4  "<TargetTypeID[-]>"
  Fault Injection Radar/1 -> radarDetections/1
  [other] -> radarDetections/Enable
  [yaw_rate] -> ROS Send IMU/4
  Clock/1 -> ROS Send Clock/1
  [RADAR] -> Bus Selector1/1
  [L1] -> ROS Send Lidar/1
  [clock] -> ROS Send Clock/Enable
  [yaw_rate] -> ROS Send Odometry/3
  [L2] -> ROS Send Lidar/2
  Constant9/1 -> Fault Injection Radar/5
  [other] -> ROS Send IMU/Enable
  [vel] -> ROS Send Velocity/Enable
  [G2] -> ROS Send Camera TL/2
  Fault Injection Radar/2 -> radarDetections/2
  [yaw_rate] -> ROS Send Velocity/2
  [image] -> ROS Send Camera TL/Enable
  Bus Selector1/1 -> Fault Injection Radar/1  "<Range[m]>"
  [Rotx] -> ROS Send IMU/1
  [velocity] -> ROS Send IMU/5
  Fault Injection Radar/3 -> radarDetections/3
  [velocity] -> ROS Send Velocity/1
  [L3] -> ROS Send Lidar/3
  Fault Injection Radar/4 -> radarDetections/4
  [R3] -> ROS Send Camera 2/1
  [image] -> ROS Send Camera 2/Enable
  [points] -> ROS Send Lidar/Enable
  [velocity] -> ROS Send Odometry/2
  Constant20/1 -> ROS Send Odometry/Enable
  [B3] -> ROS Send Camera 2/3
  [Rotz] -> ROS Send IMU/3
  [R2] -> ROS Send Camera TL/1
  [base_link_pose] -> ROS Send Odometry/1
  [L4] -> ROS Send Lidar/4
  [B2] -> ROS Send Camera TL/3
  Bus Selector1/3 -> Fault Injection Radar/3  "<Phi[deg]>"
  Bus Selector1/2 -> Fault Injection Radar/2  "<Theta[deg]>"
  [B1] -> ROS Send Camera/3
  [image] -> ROS Send Camera/Enable
  [G1] -> ROS Send Camera/2
  [R1] -> ROS Send Camera/1
  2D Orientation to Quaternion/1 -> ROS Send Goal/4
  2D Orientation to Quaternion/2 -> ROS Send Goal/5
  2D Orientation to Quaternion/3 -> ROS Send Goal/6
  2D Orientation to Quaternion/4 -> ROS Send Goal/7
  GoalOrientZ/1 -> 2D Orientation to Quaternion/1
  STATE_BMW_X5_SUV_2_rc/1 -> STATE_BMW_X5_SUV_2_bus/1
  SELF_BMW_X5_SUV_2/1 -> SELF_Demux/1(SELF)
  Radar_1/1 -> Radar_1_Demux/1(Radar)
  Radar_1_Location/1 -> Mux_Radar_1_TA/1(Location)
  Radar_1_Orientation/1 -> Mux_Radar_1_TA/2(Orientation)
  Radar_1_Range/1 -> Mux_Radar_1_TA/3(Range)
  Radar_1_NoiseAzimuthIllumination/1 -> Mux_Radar_1_TA/4(NoiseAzimuthIllumination)
  Radar_1_NoiseAziIlluType/1 -> Mux_Radar_1_TA/5(NoiseAziIlluType)
  Radar_1_NoiseElevationIllumination/1 -> Mux_Radar_1_TA/6(NoiseElevationIllumination)
  Radar_1_NoiseElevIlluType/1 -> Mux_Radar_1_TA/7(NoiseElevIlluType)
  Radar_1_NoiseAzimuthReflection/1 -> Mux_Radar_1_TA/8(NoiseAzimuthReflection)
  Radar_1_NoiseAziReflectType/1 -> Mux_Radar_1_TA/9(NoiseAziReflectType)
  Radar_1_NoiseElevationReflection/1 -> Mux_Radar_1_TA/10(NoiseElevationReflection)
  Radar_1_NoiseElevReflectType/1 -> Mux_Radar_1_TA/11(NoiseElevReflectType)
  Radar_1_NoiseRange/1 -> Mux_Radar_1_TA/12(NoiseRange)
  Radar_1_NoiseRangeType/1 -> Mux_Radar_1_TA/13(NoiseRangeType)
  Mux_Radar_1_TA/1(TA) -> Radar_1_TA/1
  PointCloudSensor_1/1 -> PointCloudSensor_1_Range_Demux/1(In1), PointCloudSensor_1_Angles_Demux/1(In2), PointCloudSensor_1_Intensity_Demux/1(In1)
  PointCloudSensor_1_Location/1 -> Mux_PointCloudSensor_1_TA/1(Location)
  PointCloudSensor_1_Orientation/1 -> Mux_PointCloudSensor_1_TA/2(Orientation)
  PointCloudSensor_1_FovAzimuth/1 -> Mux_PointCloudSensor_1_TA/3(FovAzimuth)
  PointCloudSensor_1_FovElevation/1 -> Mux_PointCloudSensor_1_TA/4(FovElevation)
  Mux_PointCloudSensor_1_TA/1(TA) -> PointCloudSensor_1_TA/1
  PointCloudSensor_2/1 -> PointCloudSensor_2_Range_Demux/1(In1), PointCloudSensor_2_Angles_Demux/1(In2), PointCloudSensor_2_Intensity_Demux/1(In1)
  PointCloudSensor_2_Location/1 -> Mux_PointCloudSensor_2_TA/1(Location)
  PointCloudSensor_2_Orientation/1 -> Mux_PointCloudSensor_2_TA/2(Orientation)
  PointCloudSensor_2_FovAzimuth/1 -> Mux_PointCloudSensor_2_TA/3(FovAzimuth)
  PointCloudSensor_2_FovElevation/1 -> Mux_PointCloudSensor_2_TA/4(FovElevation)
  Mux_PointCloudSensor_2_TA/1(TA) -> PointCloudSensor_2_TA/1
  PointCloudSensor_3/1 -> PointCloudSensor_3_Range_Demux/1(In1), PointCloudSensor_3_Angles_Demux/1(In2), PointCloudSensor_3_Intensity_Demux/1(In1)
  PointCloudSensor_3_Location/1 -> Mux_PointCloudSensor_3_TA/1(Location)
  PointCloudSensor_3_Orientation/1 -> Mux_PointCloudSensor_3_TA/2(Orientation)
  PointCloudSensor_3_FovAzimuth/1 -> Mux_PointCloudSensor_3_TA/3(FovAzimuth)
  PointCloudSensor_3_FovElevation/1 -> Mux_PointCloudSensor_3_TA/4(FovElevation)
  Mux_PointCloudSensor_3_TA/1(TA) -> PointCloudSensor_3_TA/1
  PointCloudSensor_4/1 -> PointCloudSensor_4_Range_Demux/1(In1), PointCloudSensor_4_Angles_Demux/1(In2), PointCloudSensor_4_Intensity_Demux/1(In1)
  PointCloudSensor_4_Location/1 -> Mux_PointCloudSensor_4_TA/1(Location)
  PointCloudSensor_4_Orientation/1 -> Mux_PointCloudSensor_4_TA/2(Orientation)
  PointCloudSensor_4_FovAzimuth/1 -> Mux_PointCloudSensor_4_TA/3(FovAzimuth)
  PointCloudSensor_4_FovElevation/1 -> Mux_PointCloudSensor_4_TA/4(FovElevation)
  Mux_PointCloudSensor_4_TA/1(TA) -> PointCloudSensor_4_TA/1
  Camera_1/1 -> Camera_1_CM_Demux/1(In1)
  Camera_1_Location/1 -> Mux_Camera_1_TA/1(Location)
  Camera_1_Orientation/1 -> Mux_Camera_1_TA/2(Orientation)
  Camera_1_IntensityFactorRGBMono/1 -> Mux_Camera_1_TA/3(IntensityFactorRGBMono)
  Camera_1_FoVAzimuth/1 -> Mux_Camera_1_TA/4(FoVAzimuth)
  Camera_1_FoVElevation/1 -> Mux_Camera_1_TA/5(FoVElevation)
  Camera_1_MisAlignMountPos/1 -> Mux_Camera_1_TA/6(MisAlignMountPos)
  Camera_1_MisAlignMountOrient/1 -> Mux_Camera_1_TA/7(MisAlignMountOrient)
  Mux_Camera_1_TA/1(TA) -> Camera_1_TA/1
  Camera_tl/1 -> Camera_tl_CM_Demux/1(In1)
  Camera_tl_Location/1 -> Mux_Camera_tl_TA/1(Location)
  Camera_tl_Orientation/1 -> Mux_Camera_tl_TA/2(Orientation)
  Camera_tl_IntensityFactorRGBMono/1 -> Mux_Camera_tl_TA/3(IntensityFactorRGBMono)
  Camera_tl_FoVAzimuth/1 -> Mux_Camera_tl_TA/4(FoVAzimuth)
  Camera_tl_FoVElevation/1 -> Mux_Camera_tl_TA/5(FoVElevation)
  Camera_tl_MisAlignMountPos/1 -> Mux_Camera_tl_TA/6(MisAlignMountPos)
  Camera_tl_MisAlignMountOrient/1 -> Mux_Camera_tl_TA/7(MisAlignMountOrient)
  Mux_Camera_tl_TA/1(TA) -> Camera_tl_TA/1
  HumViewCamera/1 -> HumViewCamera_CM_Demux/1(In1)
  HumViewCamera_CM_Demux/1(R) -> HumViewCamera_CM_Display/1
  HumViewCamera_CM_Demux/2(G) -> HumViewCamera_CM_Display/2
  HumViewCamera_CM_Demux/3(B) -> HumViewCamera_CM_Display/3
  HumViewCamera_Location/1 -> Mux_HumViewCamera_TA/1(Location)
  HumViewCamera_Orientation/1 -> Mux_HumViewCamera_TA/2(Orientation)
  HumViewCamera_IntensityFactorRGBMono/1 -> Mux_HumViewCamera_TA/3(IntensityFactorRGBMono)
  HumViewCamera_FoVAzimuth/1 -> Mux_HumViewCamera_TA/4(FoVAzimuth)
  HumViewCamera_FoVElevation/1 -> Mux_HumViewCamera_TA/5(FoVElevation)
  HumViewCamera_MisAlignMountPos/1 -> Mux_HumViewCamera_TA/6(MisAlignMountPos)
  HumViewCamera_MisAlignMountOrient/1 -> Mux_HumViewCamera_TA/7(MisAlignMountOrient)
  Mux_HumViewCamera_TA/1(TA) -> HumViewCamera_TA/1
  Camera_2/1 -> Camera_2_CM_Demux/1(In1)
  Camera_2_Location/1 -> Mux_Camera_2_TA/1(Location)
  Camera_2_Orientation/1 -> Mux_Camera_2_TA/2(Orientation)
  Camera_2_IntensityFactorRGBMono/1 -> Mux_Camera_2_TA/3(IntensityFactorRGBMono)
  Camera_2_FoVAzimuth/1 -> Mux_Camera_2_TA/4(FoVAzimuth)
  Camera_2_FoVElevation/1 -> Mux_Camera_2_TA/5(FoVElevation)
  Camera_2_MisAlignMountPos/1 -> Mux_Camera_2_TA/6(MisAlignMountPos)
  Camera_2_MisAlignMountOrient/1 -> Mux_Camera_2_TA/7(MisAlignMountOrient)
  Mux_Camera_2_TA/1(TA) -> Camera_2_TA/1
  Dynamics_Empty/1(State) -> STATE_BMW_X5_SUV_2_rc/1
  SELF_Demux/7(GPS lat [deg]) -> Terminator_1/1
  SELF_Demux/8(GPS long [deg]) -> Terminator_2/1
  SELF_Demux/9(GPS alt [m]) -> Terminator_3/1
  SELF_Demux/11(heading [deg]) -> Terminator_4/1

== system W06_city_highway_cs/Camera_1 ==
  Sensor : S-Function  FunctionName=sfun_Camera  Parameters=sensorID, dataWidth, dataHeight, channelsPerImage, numberOfImages, timestep  SFunctionDeploymentMode=off  EnableBusSupport=off  mask(PreScan Source Block: Camera Sensor){sensorID=6411, dataWidth=720, dataHeight=2880, channelsPerImage=3, numberOfImages=1, timestep=1/20}
      mask prompts: sensorID "Sensor ID"; dataWidth "Data width"; dataHeight "Data Height"; channelsPerImage "Channels per image"; numberOfImages "Number of images"; timestep "MATLAB timestep:"
      mask help: The Camera Sensor provides a color or monochrome image.
      mask Help: eval('openHelp(457)')
      mask Display: image(imread('CameraSensor.png'))
  Camera_1 : Outport  Tag=outport/Camera/CameraSensor  OutDataTypeStr=uint8  SampleTime=1/20
  wires:
  Sensor/1 -> Camera_1/1

== system W06_city_highway_cs/Camera_1_TA ==
  Camera_1_TA : Inport  Tag=inport/Camera_TA/CameraSensor  OutDataTypeStr=Bus: PRESCAN_CAMERASENSOR_TA  PortDimensions=1  SampleTime=1/60  BusOutputAsStruct=on
  Actuator : S-Function  FunctionName=sfun_Camera_TA  Parameters=sensorID, timestep  SFunctionDeploymentMode=off  EnableBusSupport=off  mask(Camera Sensor Test Automation){sensorID=6411, timestep=1/60}
      mask prompts: sensorID "Sensor ID"; timestep "MATLAB timestep:"
      mask help:
      | The TA Sink block updates the Test Automation variables in the Simulation.
      |
      | Note: All angles are expressed in degrees
      |
      | Remarks:
      | TIS: Drift Type:
      |   0: None
      |   1: Gaussian
      |   2: Unidirectional
      |
      | TIS: Noise Type:
      |   0: Additive
      |   1: Multiplicative
      |
      | AIR: Detection Type:
      |   0: BoundingBox
      |   1: Bounding Box Center
      |   2: CenterOfGravity
      |
      | Antenna Tx: Range
      |   -1: Infinite
      |
      | For more information, please click Help.
      mask Help: eval('openHelp(633)')
      mask Display: image(imread('TA.png'))
  wires:
  Camera_1_TA/1 -> Actuator/1

== system W06_city_highway_cs/Camera_2 ==
  Sensor : S-Function  FunctionName=sfun_Camera  Parameters=sensorID, dataWidth, dataHeight, channelsPerImage, numberOfImages, timestep  SFunctionDeploymentMode=off  EnableBusSupport=off  mask(PreScan Source Block: Camera Sensor){sensorID=6415, dataWidth=720, dataHeight=2880, channelsPerImage=3, numberOfImages=1, timestep=1/20}
      mask prompts: sensorID "Sensor ID"; dataWidth "Data width"; dataHeight "Data Height"; channelsPerImage "Channels per image"; numberOfImages "Number of images"; timestep "MATLAB timestep:"
      mask help: The Camera Sensor provides a color or monochrome image.
      mask Help: eval('openHelp(457)')
      mask Display: image(imread('CameraSensor.png'))
  Camera_2 : Outport  Tag=outport/Camera/CameraSensor  OutDataTypeStr=uint8  SampleTime=1/20
  wires:
  Sensor/1 -> Camera_2/1

== system W06_city_highway_cs/Camera_2_TA ==
  Camera_2_TA : Inport  Tag=inport/Camera_TA/CameraSensor  OutDataTypeStr=Bus: PRESCAN_CAMERASENSOR_TA  PortDimensions=1  SampleTime=1/60  BusOutputAsStruct=on
  Actuator : S-Function  FunctionName=sfun_Camera_TA  Parameters=sensorID, timestep  SFunctionDeploymentMode=off  EnableBusSupport=off  mask(Camera Sensor Test Automation){sensorID=6415, timestep=1/60}
      mask prompts: sensorID "Sensor ID"; timestep "MATLAB timestep:"
      mask help:
      | The TA Sink block updates the Test Automation variables in the Simulation.
      |
      | Note: All angles are expressed in degrees
      |
      | Remarks:
      | TIS: Drift Type:
      |   0: None
      |   1: Gaussian
      |   2: Unidirectional
      |
      | TIS: Noise Type:
      |   0: Additive
      |   1: Multiplicative
      |
      | AIR: Detection Type:
      |   0: BoundingBox
      |   1: Bounding Box Center
      |   2: CenterOfGravity
      |
      | Antenna Tx: Range
      |   -1: Infinite
      |
      | For more information, please click Help.
      mask Help: eval('openHelp(633)')
      mask Display: image(imread('TA.png'))
  wires:
  Camera_2_TA/1 -> Actuator/1

== system W06_city_highway_cs/Camera_tl ==
  Sensor : S-Function  FunctionName=sfun_Camera  Parameters=sensorID, dataWidth, dataHeight, channelsPerImage, numberOfImages, timestep  SFunctionDeploymentMode=off  EnableBusSupport=off  mask(PreScan Source Block: Camera Sensor){sensorID=6412, dataWidth=720, dataHeight=2880, channelsPerImage=3, numberOfImages=1, timestep=1/20}
      mask prompts: sensorID "Sensor ID"; dataWidth "Data width"; dataHeight "Data Height"; channelsPerImage "Channels per image"; numberOfImages "Number of images"; timestep "MATLAB timestep:"
      mask help: The Camera Sensor provides a color or monochrome image.
      mask Help: eval('openHelp(457)')
      mask Display: image(imread('CameraSensor.png'))
  Camera_tl : Outport  Tag=outport/Camera/CameraSensor  OutDataTypeStr=uint8  SampleTime=1/20
  wires:
  Sensor/1 -> Camera_tl/1
